simulink model "test"  (R2018a)
settings: Solver=VariableStepAuto  StartTime=0.0  StopTime=100  RelTol=1e-3
libraries: simulink x1
settings Model: Creator=john  LastModifiedBy=john

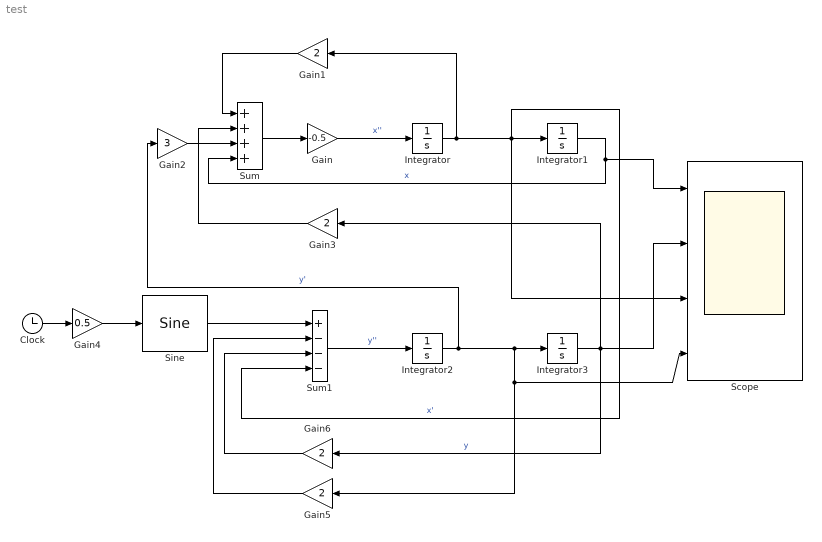
== system test ==
  Clock : Clock
  Gain : Gain  Gain=-0.5
  Gain{1,3,5..6} (4 alike) : Gain  Gain=2
  Gain2 : Gain  Gain=3
  Gain4 : Gain  Gain=0.5
  Integrator{,1..3} (4 alike) : Integrator
  Scope : Scope  NumInputPorts=4
  Sine : simulink/Lookup Tables/Sine  Formula=sin(2*pi*u)  NumDataPoints=(2^5)+1  OutputWordLength=16  InternalRulePriority=Speed
      settings: SourceProductName=Simulink
  Sum : Sum  Inputs=++++
  Sum1 : Sum  Inputs=+---
  wires:
  Integrator/1 -> Gain1/1, Scope/3, Sum1/4, Integrator1/1  "x'"
  Integrator2/1 -> Gain2/1, Scope/4, Gain5/1, Integrator3/1  "y'"
  Gain/1 -> Integrator/1  "x''"
  Gain1/1 -> Sum/1
  Sum/1 -> Gain/1
  Gain2/1 -> Sum/3
  Integrator1/1 -> Scope/1, Sum/4  "x"
  Integrator3/1 -> Scope/2, Gain6/1, Gain3/1  "y"
  Gain3/1 -> Sum/2
  Sum1/1 -> Integrator2/1  "y''"
  Clock/1 -> Gain4/1
  Gain4/1 -> Sine/1
  Sine/1 -> Sum1/1
  Gain5/1 -> Sum1/2
  Gain6/1 -> Sum1/3
